simulink model "TC_TV_Simulation"  (R2025b)
settings: Solver=FixedStepAuto  StartTime=0  StopTime=180  FixedStep=0.001  RelTol=1e-3
PostLoadFcn:
  | setup_custom_code_paths_Sim(bdroot);
settings Model: Creator=simde  LastModifiedBy=simde
settings SFSimCC: SimCustomHeaderCode=TV.h  SimUserSources=TV.c  SimUserIncludeDirs=C:\Users\simde\OneDrive\Bureau\vcu-firmware\C_code  DefaultCustomCodeDeterministicFunctions=All
settings RTWCC: RTWUseSimCustomCode=on  CustomHeaderCode=TV.h  CustomInclude=C:\Users\simde\OneDrive\Bureau\vcu-firmware\C_code  CustomSource=TV.c

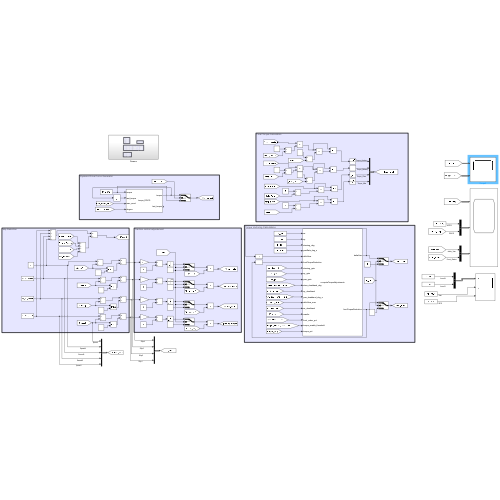
[thumbnail: Simulink's stored preview of the top-level diagram]
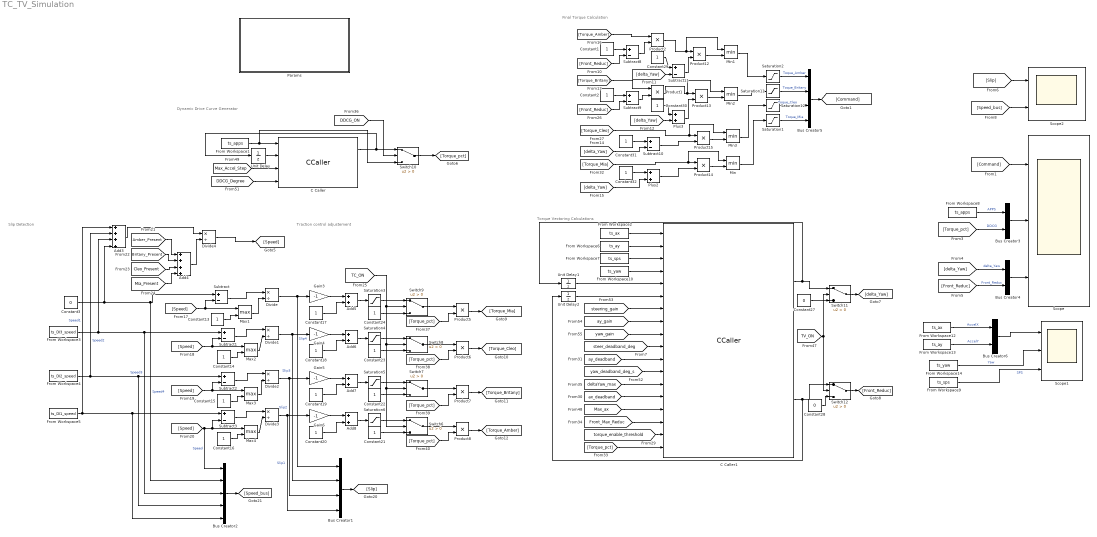
== system TC_TV_Simulation ==
  note: Traction control adjustement
  note: Slip Detection
  note: Final Torque Calculation
  note: Dynamic Drive Curve Generator
  note: Torque Vectoring Calculations
  Add3 : Sum  Inputs=++++
  Add4 : Sum  Inputs=++++
  Add{5..8} (4 alike) : Sum
  Bus Creator1 : BusCreator  Inputs=4
  Bus Creator2 : BusCreator  Inputs=5
  Bus Creator3 : BusCreator  Inputs=2
  Bus Creator4 : BusCreator  Inputs=2
  Bus Creator5 : BusCreator  Inputs=4
  Bus Creator6 : BusCreator  Inputs=2
  C Caller : CCaller  FunctionName=torque_DDCG  PortSpecificationStruct="%)30     .    : <   8    (     @         %    \"     0    !     0         %  0 \"0    $    _    07)G3F%M90  4&]R=$YA;64 4V-O<&4     26YD97@     5'EP90      4VEZ90      27-';&]B86P   X    X    !@    @    $          4    (     0    8    !         !     &    =&]R<75E   .    .     8    (    !          %    \"     $    &     0         0    !@   '1O<G%U90  #@   $     &    \"     0         !0    @    !   ...(+2178 chars)"
  C Caller1 : CCaller  FunctionName=computeTorqueAdjustments  PortSpecificationStruct="%)30     .    R!\\   8    (     @         %    \"    !(    !     0         %  0 \"0    $    _    07)G3F%M90  4&]R=$YA;64 4V-O<&4     26YD97@     5'EP90      4VEZ90      27-';&]B86P   X    P    !@    @    $          4    (     0    (    !         !   @!A>   #@   #     &    \"     0         !0    @    !     @    $         $  \" &%X   .    .     8    (    !          %    \"     $    %     0         0 ...(+10597 chars)"
  Constant{1..2,13..24,29..32} (18 alike) : Constant
  Constant27 : Constant  Value=0
  Constant28 : Constant  Value=0
  Constant3 : Constant  Value=0  OutDataTypeStr=single
  Divide{,1..3} (4 alike) : Product  Inputs=*/
  Divide4 : Product  Inputs=*/  OutDataTypeStr=single
  From Workspace1 : FromWorkspace  VariableName=ts_apps
  From Workspace10 : FromWorkspace  VariableName=ts_yaw
  From Workspace12 : FromWorkspace  VariableName=ts_ax
  From Workspace13 : FromWorkspace  VariableName=ts_ay
  From Workspace14 : FromWorkspace  VariableName=ts_yaw
  From Workspace2 : FromWorkspace  VariableName=ts_ax
  From Workspace3 : FromWorkspace  VariableName=ts_DI3_speed
  From Workspace4 : FromWorkspace  VariableName=ts_DI2_speed
  From Workspace5 : FromWorkspace  VariableName=ts_DI1_speed
  From Workspace6 : FromWorkspace  VariableName=ts_ay
  From Workspace7 : FromWorkspace  VariableName=ts_sps
  From Workspace8 : FromWorkspace  VariableName=ts_apps
  From Workspace9 : FromWorkspace  VariableName=ts_sps
  Gain{3..6} (4 alike) : Gain  Gain=-1
  Max{1..4} (4 alike) : MinMax  Function=max  Inputs=2
  Min{,1..3} (4 alike) : MinMax  Inputs=2
  Params : Subsystem
  Plus2 : Sum
  Plus3 : Sum
  Product{1..2,5..8,12..15} (10 alike) : Product
  Saturation{1..2,11..12} (4 alike) : Saturate  UpperLimit=100  LowerLimit=0
  Saturation{3..6} (4 alike) : Saturate  UpperLimit=1  LowerLimit=0
  Scope : Scope  NumInputPorts=3
      settings: ActiveDisplayYMinimum=-12.499783515930172  ActiveDisplayYMaximum=112.49805164337158
  Scope1 : Scope  NumInputPorts=3
      settings: ActiveDisplayYMinimum=-1.5983438789844513  ActiveDisplayYMaximum=1.5887048542499542
  Scope2 : Scope  NumInputPorts=2
      settings: ActiveDisplayYMinimum=-1.4776564015060158  ActiveDisplayYMaximum=2.4552166913179168  DataLoggingVariableName=ScopeData2
  Subtract{,1..3,8..11} (8 alike) : Sum  Inputs=+-
  Switch{6..12} (7 alike) : Switch  Criteria=u2 > Threshold  SaturateOnIntegerOverflow=off  InputSameDT=off
  Unit Delay : UnitDelay  SampleTime=-1  HasFrameUpgradeWarning=on
  Unit Delay1 : UnitDelay  SampleTime=-1  HasFrameUpgradeWarning=on
  Unit Delay2 : UnitDelay  SampleTime=-1  HasFrameUpgradeWarning=on
  wires:
  Product8/1 -> [Torque_Amber]
  Divide2/1 -> Bus Creator1/3, Gain5/1  "Slip2"
  Divide3/1 -> Bus Creator1/4, Gain6/1  "Slip1"
  Saturation4/1 -> Switch8/1
  Divide/1 -> Bus Creator1/1, Gain3/1  "Slip4"
  [Torque_pct] -> Product6/2
  Switch9/1 -> Product5/1
  Add6/1 -> Saturation4/1
  Subtract/1 -> Divide/1
  Constant22/1 -> Switch7/3
  Constant14/1 -> Max2/2
  Subtract1/1 -> Divide1/1
  Max2/1 -> Divide1/2
  [Torque_pct] -> Product5/2
  [Speed] -> Max2/1, Subtract1/2
  Product5/1 -> [Torque_Mia]
  Add3/1 -> Divide4/1
  Constant13/1 -> Max1/2
  Gain5/1 -> Add7/1
  Constant19/1 -> Add7/2
  Max1/1 -> Divide/2
  Saturation5/1 -> Switch7/1
  Divide1/1 -> Bus Creator1/2, Gain4/1  "Slip3"
  [TC_ON] -> Switch9/2, Switch8/2, Switch7/2, Switch6/2
  [Speed] -> Max1/1, Subtract/2
  [Mia_Present] -> Add4/4
  Switch7/1 -> Product7/1
  Gain3/1 -> Add5/1
  Constant24/1 -> Switch9/3
  Saturation6/1 -> Switch6/1
  Constant18/1 -> Add6/2
  Gain4/1 -> Add6/1
  Constant16/1 -> Max4/2
  Max4/1 -> Divide3/2
  Subtract3/1 -> Divide3/1
  [Speed] -> Bus Creator2/1, Max4/1, Subtract3/2  "Speed"
  [Cleo_Present] -> Add4/3
  [Torque_pct] -> Product8/2
  Add4/1 -> Divide4/2
  Gain6/1 -> Add8/1
  Subtract2/1 -> Divide2/1
  [Speed] -> Max3/1, Subtract2/2
  [Torque_pct] -> Product7/2
  Max3/1 -> Divide2/2
  Add8/1 -> Saturation6/1
  Constant21/1 -> Switch6/3
  Constant3/1 -> Add3/4, Bus Creator2/2, Subtract/1  "Speed4"
  Product6/1 -> [Torque_Cleo]
  Constant23/1 -> Switch8/3
  [Britany_Present] -> Add4/2
  Switch8/1 -> Product6/1
  Product7/1 -> [Torque_Britany]
  Add7/1 -> Saturation5/1
  Saturation3/1 -> Switch9/1
  Add5/1 -> Saturation3/1
  Switch6/1 -> Product8/1
  Constant15/1 -> Max3/2
  Constant20/1 -> Add8/2
  [Amber_Present] -> Add4/1
  Constant17/1 -> Add5/2
  Divide4/1 -> [Speed]
  From Workspace3/1 -> Add3/3, Bus Creator2/3, Subtract1/1  "Speed3"
  From Workspace4/1 -> Add3/2, Bus Creator2/4, Subtract2/1  "Speed2"
  From Workspace5/1 -> Add3/1, Bus Creator2/5, Subtract3/1  "Speed1"
  Bus Creator1/1 -> [Slip]
  Bus Creator2/1 -> [Speed_bus]
  [Command] -> Scope/1
  Bus Creator4/1 -> Scope/3
  [delta_Yaw] -> Bus Creator4/1  "delta_Yaw"
  [Front_Reduc] -> Bus Creator4/2  "Front_Reduc"
  Saturation2/1 -> Bus Creator5/1  "Toque_Amber"
  [delta_Yaw] -> Plus3/2
  Constant1/1 -> Subtract8/1
  [Torque_Amber] -> Product2/1
  Subtract11/1 -> Product12/2
  Constant31/1 -> Subtract10/1
  Bus Creator5/1 -> [Command]
  [Torque_Britany] -> Product1/1
  [delta_Yaw] -> Plus2/2
  [delta_Yaw] -> Subtract10/2
  Constant29/1 -> Subtract11/1
  Plus2/1 -> Product14/2
  Constant30/1 -> Plus3/1
  Product1/1 -> Min2/1, Product13/1
  Constant32/1 -> Plus2/1
  Saturation12/1 -> Bus Creator5/3  "Toque_Cleo"
  Product2/1 -> Min1/1, Product12/1
  [delta_Yaw] -> Subtract11/2
  Subtract8/1 -> Product2/2
  [Torque_Mia] -> Min/1, Product14/1
  [Torque_Cleo] -> Min3/1, Product15/1
  [Front_Reduc] -> Subtract9/2
  Subtract10/1 -> Product15/2
  Constant2/1 -> Subtract9/1
  [Front_Reduc] -> Subtract8/2
  Saturation11/1 -> Bus Creator5/2  "Toque_Britany"
  Saturation1/1 -> Bus Creator5/4  "Toque_Mia"
  Subtract9/1 -> Product1/2
  Plus3/1 -> Product13/2
  C Caller/1 -> Unit Delay/1, Switch10/1
  [DDCG_Degree] -> C Caller/4
  Switch10/1 -> [Torque_pct]
  From Workspace1/1 -> C Caller/1, Switch10/3
  Unit Delay/1 -> C Caller/2
  [DDCG_ON] -> Switch10/2
  [Max_Accel_Step] -> C Caller/3
  [yaw_deadband_deg_s] -> C Caller1/12
  Switch11/1 -> [delta_Yaw]
  [TV_ON] -> Switch12/2, Switch11/2
  C Caller1/2 -> Switch12/1, Unit Delay2/1
  [steering_gain] -> C Caller1/7
  Switch12/1 -> [Front_Reduc]
  Constant27/1 -> Switch11/3
  C Caller1/1 -> Unit Delay1/1, Switch11/1
  Unit Delay1/1 -> C Caller1/5
  [steer_deadband_deg] -> C Caller1/10
  Constant28/1 -> Switch12/3
  [yaw_gain] -> C Caller1/9
  [Max_ax] -> C Caller1/15
  [Torque_pct] -> C Caller1/18
  Unit Delay2/1 -> C Caller1/6
  [ay_gain] -> C Caller1/8
  [ay_deadband] -> C Caller1/11
  [torque_enable_threshold] -> C Caller1/17
  [deltaYaw_max] -> C Caller1/13
  [ax_deadband] -> C Caller1/14
  [Front_Max_Reduc] -> C Caller1/16
  From Workspace10/1 -> C Caller1/4
  From Workspace7/1 -> C Caller1/3
  From Workspace6/1 -> C Caller1/2
  From Workspace2/1 -> C Caller1/1
  From Workspace13/1 -> Bus Creator6/2  "AccelY"
  From Workspace12/1 -> Bus Creator6/1  "AccelX"
  Bus Creator6/1 -> Scope1/1
  From Workspace14/1 -> Scope1/2  "Yaw"
  [Slip] -> Scope2/1
  [Speed_bus] -> Scope2/2
  [Torque_pct] -> Bus Creator3/2  "DDCG"
  Bus Creator3/1 -> Scope/2
  From Workspace8/1 -> Bus Creator3/1  "APPS"
  From Workspace9/1 -> Scope1/3  "SPS"
  Product14/1 -> Min/2
  Product15/1 -> Min3/2
  Product13/1 -> Min2/2
  Product12/1 -> Min1/2
  Min/1 -> Saturation1/1
  Min3/1 -> Saturation12/1
  Min2/1 -> Saturation11/1
  Min1/1 -> Saturation2/1

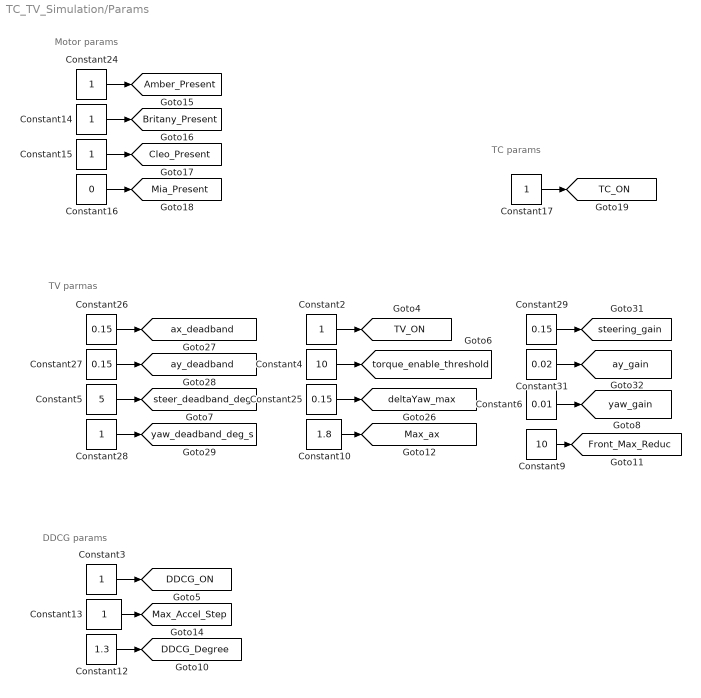
== system TC_TV_Simulation/Params ==
  note: Motor params
  note: TV parmas
  note: TC params
  note: DDCG params
  Constant10 : Constant  Value=1.8  OutDataTypeStr=single
  Constant12 : Constant  Value=1.3  OutDataTypeStr=single
  Constant13 : Constant  OutDataTypeStr=single
  Constant{2..3,14..15,17,24} (6 alike) : Constant
  Constant16 : Constant  Value=0
  Constant{25..27,29} (4 alike) : Constant  Value=0.15  OutDataTypeStr=single
  Constant28 : Constant  OutDataTypeStr=single
  Constant31 : Constant  Value=0.02  OutDataTypeStr=single
  Constant4 : Constant  Value=10  OutDataTypeStr=single
  Constant5 : Constant  Value=5  OutDataTypeStr=single
  Constant6 : Constant  Value=0.01  OutDataTypeStr=single
  Constant9 : Constant  Value=10  OutDataTypeStr=single
  tag scope: Amber_Present=global, Britany_Present=global, Cleo_Present=global, DDCG_Degree=global, DDCG_ON=global, Front_Max_Reduc=global, Max_Accel_Step=global, Max_ax=global, Mia_Present=global, TC_ON=global, TV_ON=global, ax_deadband=global, ay_deadband=global, ay_gain=global, deltaYaw_max=global, steer_deadband_deg=global, steering_gain=global, torque_enable_threshold=global, yaw_deadband_deg_s=global, yaw_gain=global
  wires:
  Constant28/1 -> [yaw_deadband_deg_s]
  Constant26/1 -> [ax_deadband]
  Constant10/1 -> [Max_ax]
  Constant15/1 -> [Cleo_Present]
  Constant13/1 -> [Max_Accel_Step]
  Constant2/1 -> [TV_ON]
  Constant14/1 -> [Britany_Present]
  Constant29/1 -> [steering_gain]
  Constant24/1 -> [Amber_Present]
  Constant5/1 -> [steer_deadband_deg]
  Constant31/1 -> [ay_gain]
  Constant6/1 -> [yaw_gain]
  Constant9/1 -> [Front_Max_Reduc]
  Constant25/1 -> [deltaYaw_max]
  Constant17/1 -> [TC_ON]
  Constant4/1 -> [torque_enable_threshold]
  Constant12/1 -> [DDCG_Degree]
  Constant16/1 -> [Mia_Present]
  Constant3/1 -> [DDCG_ON]
  Constant27/1 -> [ay_deadband]
